simulink model "master_Hinf_discrete_sys"  (R2015a)
settings: Solver=ode45  SolverMode=SingleTasking  StartTime=0.0  StopTime=10.0  RelTol=1e-3
values from neighbouring files (symbols this model uses):
  A = dsys.a    [master_Hinf.m]
  B = dsys.b    [master_Hinf.m]
  C = dsys.c    [master_Hinf.m]
  D = dsys.d    [master_Hinf.m]
  K = K(1:2)    [master_Hinf.m]
  Ts = 0.001    [master_Hinf.m]
settings Model: Creator=enrico-giordano  LastModifiedBy=enrico-giordano
settings OptimizationCC: BlockReduction=off  BooleanDataType=off
settings DebuggingCC: SaveWithParameterizedLinksMsg=none  UnderspecifiedInitializationDetection=Classic  MergeDetectMultiDrivingBlocksExec=none  SignalResolutionControl=TryResolveAllWithWarning
settings HardwareCC: TargetUnknown=on

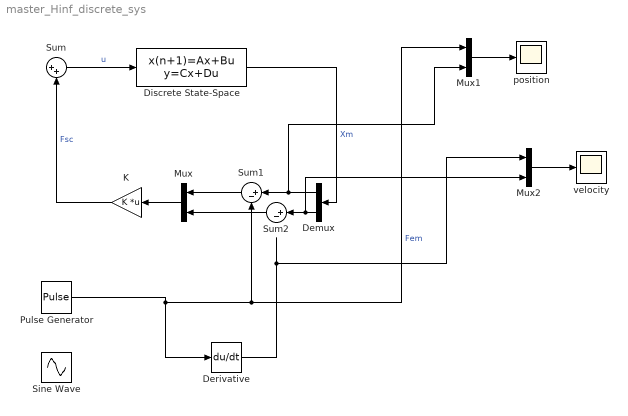
== system master_Hinf_discrete_sys ==
  Demux : Demux  Outputs=2
  Derivative : Derivative
  Discrete State-Space : DiscreteStateSpace  A=A  B=B  C=C  D=D  SampleTime=Ts
  K : Gain  Gain=K  Multiplication=Matrix(K*u)
  Mux : Mux  Inputs=2
  Mux1 : Mux  Inputs=2
  Mux2 : Mux  Inputs=2
  Pulse Generator : DiscretePulseGenerator  PulseType=Time based  PulseWidth=50
  Sine Wave : Sin  Amplitude=10  SampleTime=0
  Sum : Sum  Inputs=|++
  Sum1 : Sum  Inputs=|+-
  Sum2 : Sum  Inputs=|+-
  position : Scope
      settings: TimeRange=10  YMin=-0.6000000000000001  YMax=0.2
  velocity : Scope
      settings: TimeRange=10  YMin=-0.6000000000000001  YMax=0.2
  wires:
  Sum/1 -> Discrete State-Space/1  "u"
  Discrete State-Space/1 -> Demux/1  "Xm"
  K/1 -> Sum/2  "Fsc"
  Mux/1 -> K/1
  Demux/1 -> Mux1/2, Sum1/1
  Sum1/1 -> Mux/1
  Pulse Generator/1 -> Derivative/1, Sum1/2, Mux1/1  "Fem"
  Demux/2 -> Mux2/2, Sum2/1
  Mux1/1 -> position/1
  Sum2/1 -> Mux/2
  Derivative/1 -> Mux2/1
  Mux2/1 -> velocity/1
